simulink model "mod01"  (R2012b)
settings: Solver=ode45  StartTime=0.0  StopTime=500  RelTol=1e-3
values from neighbouring files (symbols this model uses):
  Q10 = 1.5e-4    (= 0.00015)    [semestralka_1.m]    (also in semestralka_2.m; semestralka_2druha.m)
settings Model: Creator=NTB  LastModifiedBy=NTB

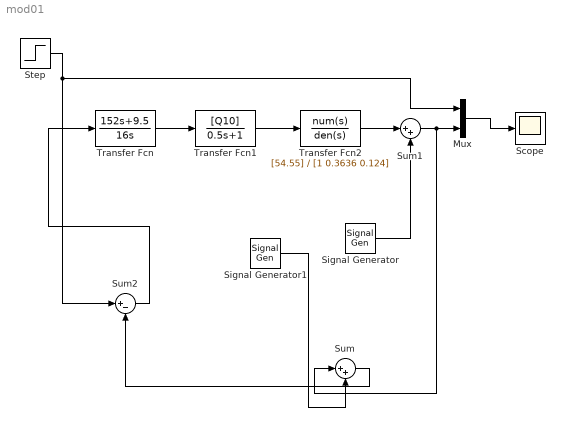
== system mod01 ==
  Mux : Mux  Inputs=2
  Scope : Scope
  Signal Generator : SignalGenerator  Amplitude=0.01  Frequency=50  VectorParams1D=off
  Signal Generator1 : SignalGenerator  Amplitude=0  Frequency=0.1
  Step : Step  After=0.5  SampleTime=0
  Sum : Sum  Inputs=|++
  Sum1 : Sum  Inputs=|++
  Sum2 : Sum  Inputs=|+-
  Transfer Fcn : TransferFcn  Numerator=[152 9.5]  Denominator=[16 0]
  Transfer Fcn1 : TransferFcn  Numerator=[Q10]  Denominator=[0.5 1]
  Transfer Fcn2 : TransferFcn  Numerator=[54.55]  Denominator=[1 0.3636 0.124]
  wires:
  Mux/1 -> Scope/1
  Sum1/1 -> Sum/1, Mux/2
  Transfer Fcn2/1 -> Sum1/1
  Transfer Fcn1/1 -> Transfer Fcn2/1
  Transfer Fcn/1 -> Transfer Fcn1/1
  Sum2/1 -> Transfer Fcn/1
  Step/1 -> Mux/1, Sum2/1
  Signal Generator/1 -> Sum1/2
  Sum/1 -> Sum2/2
  Signal Generator1/1 -> Sum/2
